simulink model "sim_ssmid"  (R2013a)
settings: Solver=ode45  StartTime=0.0  StopTime=15  RelTol=1e-3
libraries: simulink x1
settings Model: Creator=Aleksandr  LastModifiedBy=Aleksandr

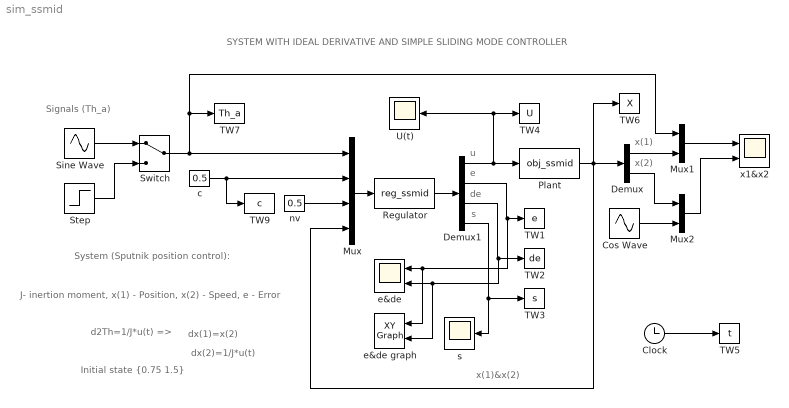
== system sim_ssmid ==
  note: Initial state {0.75 1.5}
  note: SYSTEM WITH IDEAL DERIVATIVE AND SIMPLE SLIDING MODE CONTROLLER
  note: dx(2)=1/J*u(t)
  note: dx(1)=x(2)
  note: d2Th=1/J*u(t) =>
  note: System (Sputnik position control):
  note: J- inertion moment,
      | x(1) - Position, x(2) - Speed,
      | e - Error
  note: s
  note: Signals (Th_a)
  note: x(1)&x(2)
  note: de
  note: e
  note: u
  note: x(2)
  note: x(1)
  " Switch" : ManualSwitch
  Clock : Clock
      settings: Decimation=15
  Cos Wave : Sin  Phase=pi/2  SampleTime=0
  Demux : Demux  Outputs=2
  Demux1 : Demux
  Mux : Mux
  Mux1 : Mux  Inputs=2
  Mux2 : Mux  Inputs=2
  Plant : S-Function  FunctionName=obj_ssmid  EnableBusSupport=off
  Regulator : S-Function  FunctionName=reg_ssmid  EnableBusSupport=off
  Sine Wave : Sin  SampleTime=0
  Step : Step  SampleTime=0
  TW1 : ToWorkspace  VariableName=e  SampleTime=-1
  TW2 : ToWorkspace  VariableName=de  SampleTime=-1
  TW3 : ToWorkspace  VariableName=s  SampleTime=-1
  TW4 : ToWorkspace  VariableName=U  SampleTime=-1
  TW5 : ToWorkspace  VariableName=t  SampleTime=-1
  TW6 : ToWorkspace  VariableName=X  SampleTime=-1
  TW7 : ToWorkspace  VariableName=Th_a  SampleTime=-1
  TW9 : ToWorkspace  VariableName=c  SampleTime=-1
  U(t) : Scope
  c : Constant  Value=0.5
  e&de : Scope  NumInputPorts=2
      settings: TimeRange=20  YMin=-5~-5  YMax=5~5
  e&de graph : simulink/Sinks/XY Graph  xmin=-1  xmax=2  ymin=-0.75  ymax=1.5  st=-1
  nv : Constant  Value=0.5
  s : Scope
      settings: SaveName=ScopeData3
  x1&x2 : Scope  NumInputPorts=2
      settings: TimeRange=20  YMin=-5~-5  YMax=5~5  SaveName=ScopeData2
  wires:
  " Switch"/1 -> Mux/1, TW7/1, Mux1/1
  Sine Wave/1 -> " Switch"/1
  Step/1 -> " Switch"/2
  c/1 -> Mux/2, TW9/1
  Mux/1 -> Regulator/1
  Regulator/1 -> Demux1/1
  Demux1/1 -> TW4/1, U(t)/1, Plant/1
  Demux1/2 -> e&de graph/1, e&de/1, TW1/1
  Demux1/3 -> e&de graph/2, e&de/2, TW2/1
  Demux1/4 -> s/1, TW3/1
  Plant/1 -> Mux/4, Demux/1, TW6/1
  Demux/1 -> Mux1/2
  Demux/2 -> Mux2/1
  Mux1/1 -> x1&x2/1
  Mux2/1 -> x1&x2/2
  Clock/1 -> TW5/1
  nv/1 -> Mux/3
  Cos Wave/1 -> Mux2/2
